simulink model "RL_Runcontrol"  (R2024b)
settings: Solver=VariableStepAuto  StartTime=0.0  StopTime=60  RelTol=1e-3
libraries: simulink x2, rllib x1, Solver_SF x1
settings Model: Creator=Administrator  LastModifiedBy=Administrator

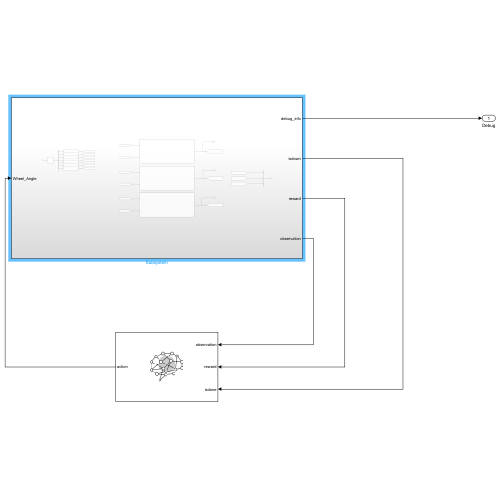
[thumbnail: Simulink's stored preview of the top-level diagram]
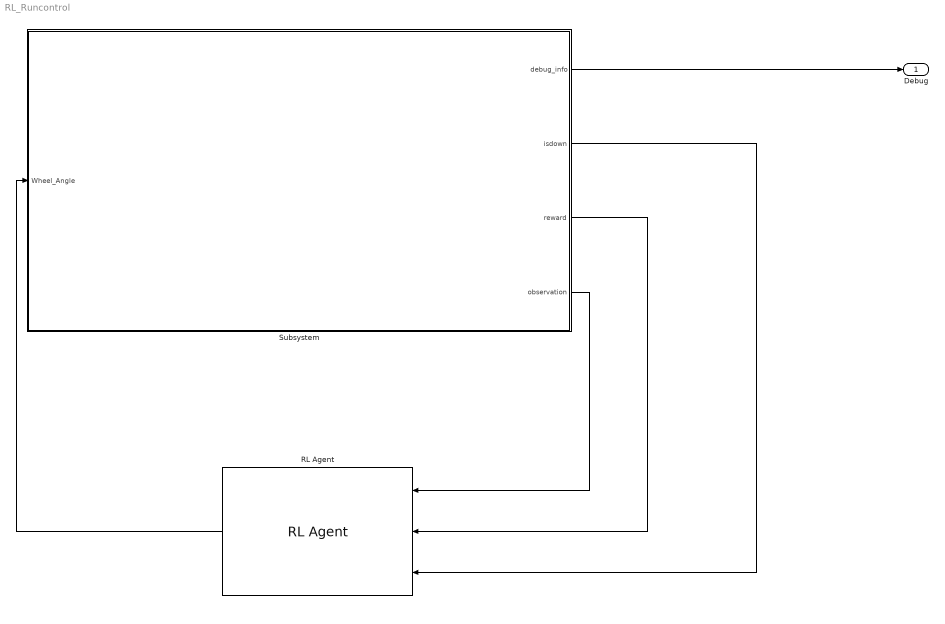
== system RL_Runcontrol ==
  RL Agent : rllib/RL Agent  Agent=agent  ExternalActionAsInput=off  ProvideLastAction=off  ProvideCumRwd=off  TreatAsDirectFeedthrough=on  UseStrictObservationDataTypes=off
  Subsystem : Subsystem
  Debug : Outport
  wires:
  RL Agent/1 -> Subsystem/1(Wheel_Angle)
  Subsystem/4(observation) -> RL Agent/1
  Subsystem/3(reward) -> RL Agent/2
  Subsystem/2(isdown) -> RL Agent/3
  Subsystem/1(debug_info) -> Debug/1

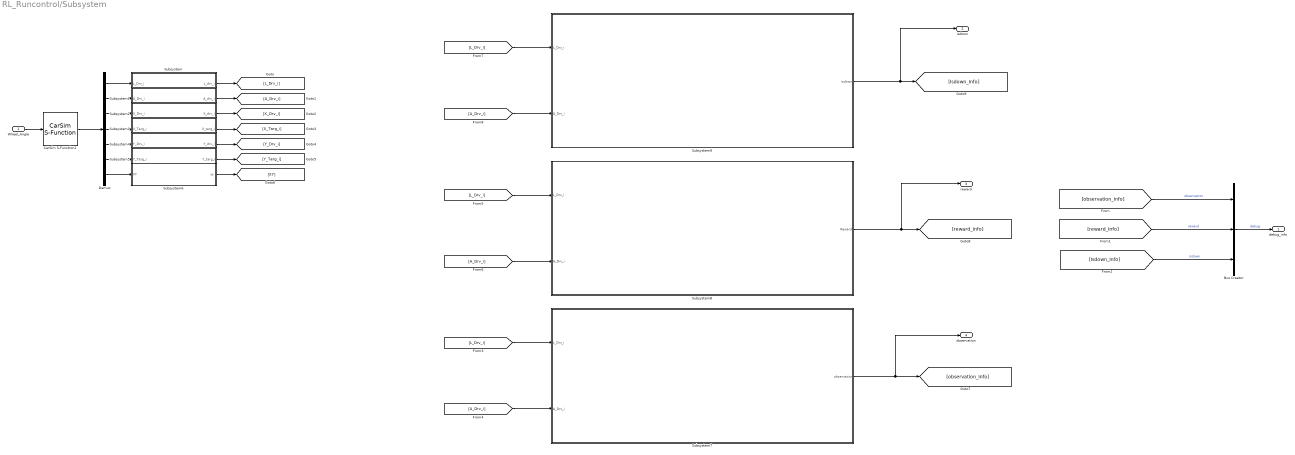
== system RL_Runcontrol/Subsystem ==
  Wheel_Angle : Inport
  Bus Creator : BusCreator  Inputs=3
  CarSim S-Function1 : Solver_SF/CarSim S-Function  Priority=1  SIMFILE=simfile.sim  Run_RTs=off  vs_state_ind=Run  StopMode_ind=Vehicle Model
  Demux : Demux  Outputs=[3 3 3 3 3 3 2]
  Subsystem : Subsystem
  Subsystem1 : Subsystem
  Subsystem2 : Subsystem
  Subsystem3 : Subsystem
  Subsystem4 : Subsystem
  Subsystem5 : Subsystem
  Subsystem6 : Subsystem
  Subsystem7 : Subsystem
  Subsystem8 : Subsystem
  Subsystem9 : Subsystem
  debug_info : Outport
  isdown : Outport  Port=2
  reward : Outport  Port=3
  observation : Outport  Port=4
  wires:
  CarSim S-Function1/1 -> Demux/1
  Wheel_Angle/1 -> CarSim S-Function1/1
  Demux/1 -> Subsystem/1(L_Drv_i)
  Demux/2 -> Subsystem1/1(A_Drv_i)
  Demux/3 -> Subsystem2/1(X_Drv_i)
  Demux/4 -> Subsystem3/1(X_Targ_i)
  Demux/5 -> Subsystem4/1(Y_Drv_i)
  Demux/6 -> Subsystem5/1(Y_Targ_i)
  Demux/7 -> Subsystem6/1(XY)
  Subsystem/1(L_drv_i) -> [L_Drv_i]
  Subsystem1/1(A_drv_i) -> [A_Drv_i]
  Subsystem2/1(X_drv_i) -> [X_Drv_i]
  Subsystem3/1(X_targ_i) -> [X_Targ_i]
  Subsystem4/1(Y_drv_i) -> [Y_Drv_i]
  Subsystem5/1(Y_targ_i) -> [Y_Targ_i]
  Subsystem6/1(xy) -> [XY]
  Subsystem7/1(observation) -> observation/1, [observation_Info]
  Subsystem8/1(Reward) -> reward/1, [reward_Info]
  Subsystem9/1(isdown) -> isdown/1, [Isdown_Info]
  [Isdown_Info] -> Bus Creator/3  "isdown"
  [reward_Info] -> Bus Creator/2  "reward"
  [observation_Info] -> Bus Creator/1  "observation"
  Bus Creator/1 -> debug_info/1  "debug"
  [L_Drv_i] -> Subsystem7/1(L_Drv_i)
  [A_Drv_i] -> Subsystem7/2(A_Drv_i)
  [A_Drv_i] -> Subsystem8/2(A_Drv_i)
  [L_Drv_i] -> Subsystem8/1(L_Drv_i)
  [L_Drv_i] -> Subsystem9/1(L_Drv_i)
  [A_Drv_i] -> Subsystem9/2(A_Drv_i)

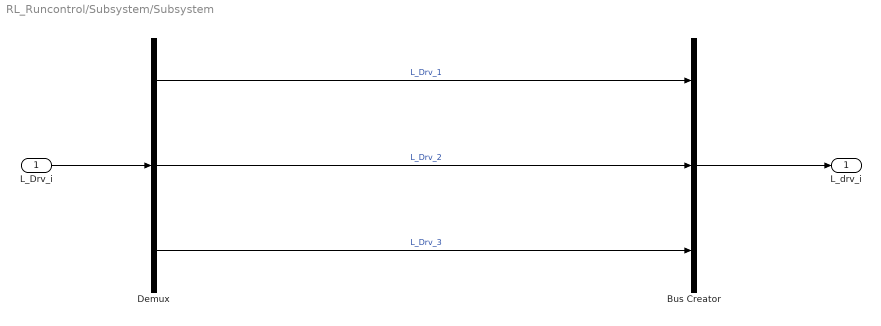
== system RL_Runcontrol/Subsystem/Subsystem ==
  L_Drv_i : Inport
  Bus Creator : BusCreator  Inputs=3
  Demux : Demux  Outputs=3
  L_drv_i : Outport
  wires:
  L_Drv_i/1 -> Demux/1
  Demux/3 -> Bus Creator/3  "L_Drv_3"
  Demux/2 -> Bus Creator/2  "L_Drv_2"
  Demux/1 -> Bus Creator/1  "L_Drv_1"
  Bus Creator/1 -> L_drv_i/1

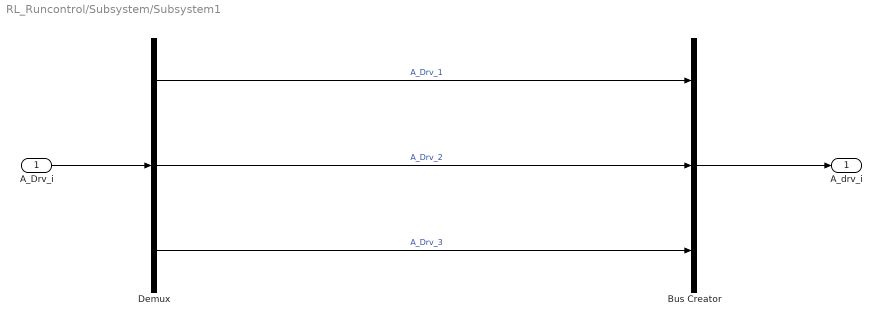
== system RL_Runcontrol/Subsystem/Subsystem1 ==
  A_Drv_i : Inport
  Bus Creator : BusCreator  Inputs=3
  Demux : Demux  Outputs=3
  A_drv_i : Outport
  wires:
  Bus Creator/1 -> A_drv_i/1
  Demux/1 -> Bus Creator/1  "A_Drv_1"
  Demux/2 -> Bus Creator/2  "A_Drv_2"
  Demux/3 -> Bus Creator/3  "A_Drv_3"
  A_Drv_i/1 -> Demux/1

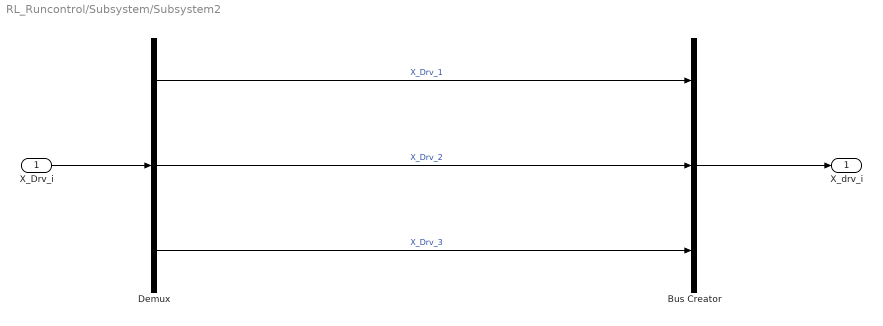
== system RL_Runcontrol/Subsystem/Subsystem2 ==
  X_Drv_i : Inport
  Bus Creator : BusCreator  Inputs=3
  Demux : Demux  Outputs=3
  X_drv_i : Outport
  wires:
  X_Drv_i/1 -> Demux/1
  Demux/3 -> Bus Creator/3  "X_Drv_3"
  Demux/2 -> Bus Creator/2  "X_Drv_2"
  Demux/1 -> Bus Creator/1  "X_Drv_1"
  Bus Creator/1 -> X_drv_i/1

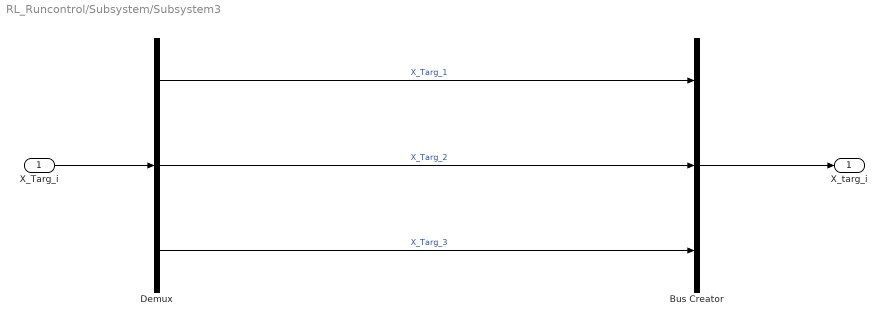
== system RL_Runcontrol/Subsystem/Subsystem3 ==
  X_Targ_i : Inport
  Bus Creator : BusCreator  Inputs=3
  Demux : Demux  Outputs=3
  X_targ_i : Outport
  wires:
  Bus Creator/1 -> X_targ_i/1
  Demux/1 -> Bus Creator/1  "X_Targ_1"
  Demux/2 -> Bus Creator/2  "X_Targ_2"
  Demux/3 -> Bus Creator/3  "X_Targ_3"
  X_Targ_i/1 -> Demux/1

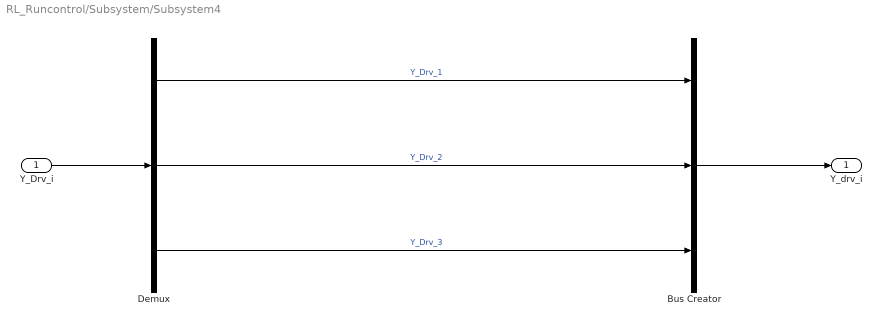
== system RL_Runcontrol/Subsystem/Subsystem4 ==
  Y_Drv_i : Inport
  Bus Creator : BusCreator  Inputs=3
  Demux : Demux  Outputs=3
  Y_drv_i : Outport
  wires:
  Y_Drv_i/1 -> Demux/1
  Demux/3 -> Bus Creator/3  "Y_Drv_3"
  Demux/2 -> Bus Creator/2  "Y_Drv_2"
  Demux/1 -> Bus Creator/1  "Y_Drv_1"
  Bus Creator/1 -> Y_drv_i/1

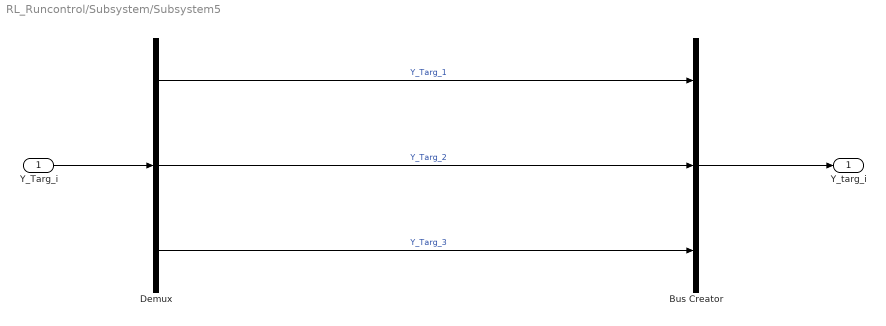
== system RL_Runcontrol/Subsystem/Subsystem5 ==
  Y_Targ_i : Inport
  Bus Creator : BusCreator  Inputs=3
  Demux : Demux  Outputs=3
  Y_targ_i : Outport
  wires:
  Bus Creator/1 -> Y_targ_i/1
  Demux/1 -> Bus Creator/1  "Y_Targ_1"
  Demux/2 -> Bus Creator/2  "Y_Targ_2"
  Demux/3 -> Bus Creator/3  "Y_Targ_3"
  Y_Targ_i/1 -> Demux/1

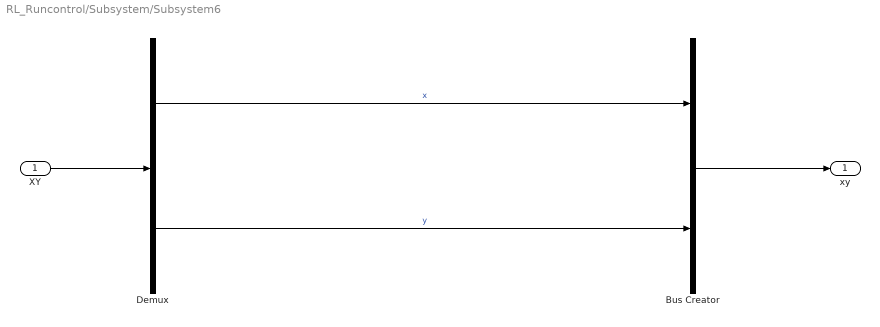
== system RL_Runcontrol/Subsystem/Subsystem6 ==
  XY : Inport
  Bus Creator : BusCreator  Inputs=2
  Demux : Demux  Outputs=2
  xy : Outport
  wires:
  XY/1 -> Demux/1
  Demux/2 -> Bus Creator/2  "y"
  Demux/1 -> Bus Creator/1  "x"
  Bus Creator/1 -> xy/1

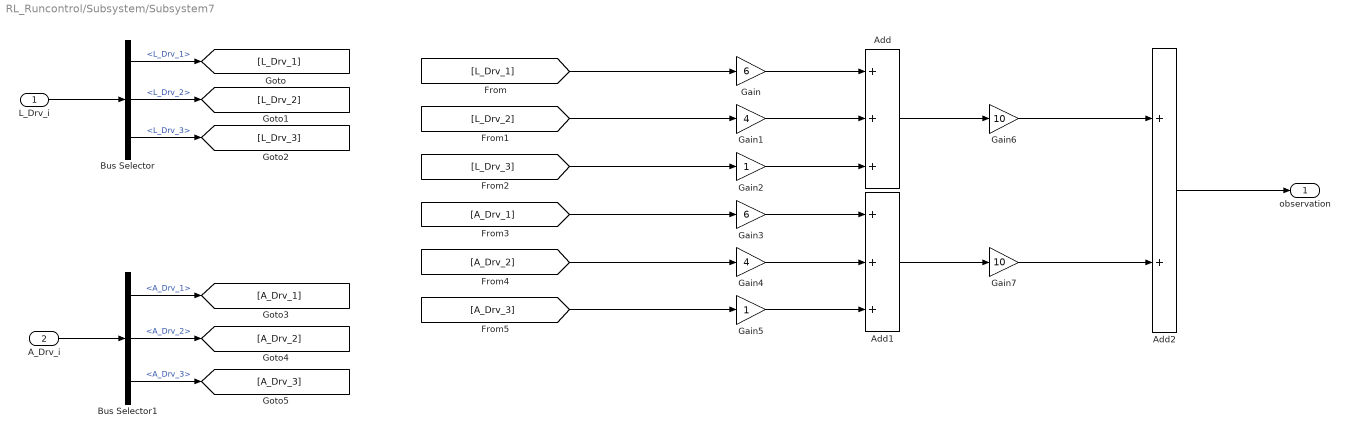
== system RL_Runcontrol/Subsystem/Subsystem7 ==
  L_Drv_i : Inport
  A_Drv_i : Inport  Port=2
  Add : Sum  Inputs=+++
  Add1 : Sum  Inputs=+++
  Add2 : Sum
  Bus Selector : BusSelector  OutputSignals=L_Drv_1,L_Drv_2,L_Drv_3
  Bus Selector1 : BusSelector  OutputSignals=A_Drv_1,A_Drv_2,A_Drv_3
  Gain : Gain  Gain=6
  Gain1 : Gain  Gain=4
  Gain2 : Gain
  Gain3 : Gain  Gain=6
  Gain4 : Gain  Gain=4
  Gain5 : Gain
  Gain6 : Gain  Gain=10
  Gain7 : Gain  Gain=10
  observation : Outport
  wires:
  L_Drv_i/1 -> Bus Selector/1
  A_Drv_i/1 -> Bus Selector1/1
  Bus Selector/1 -> [L_Drv_1]  "<L_Drv_1>"
  Bus Selector/2 -> [L_Drv_2]  "<L_Drv_2>"
  Bus Selector/3 -> [L_Drv_3]  "<L_Drv_3>"
  Bus Selector1/1 -> [A_Drv_1]  "<A_Drv_1>"
  Bus Selector1/2 -> [A_Drv_2]  "<A_Drv_2>"
  Bus Selector1/3 -> [A_Drv_3]  "<A_Drv_3>"
  [L_Drv_1] -> Gain/1
  [L_Drv_2] -> Gain1/1
  [L_Drv_3] -> Gain2/1
  [A_Drv_1] -> Gain3/1
  [A_Drv_2] -> Gain4/1
  [A_Drv_3] -> Gain5/1
  Gain/1 -> Add/1
  Gain1/1 -> Add/2
  Gain2/1 -> Add/3
  Gain3/1 -> Add1/1
  Gain4/1 -> Add1/2
  Gain5/1 -> Add1/3
  Add/1 -> Gain6/1
  Add1/1 -> Gain7/1
  Gain6/1 -> Add2/1
  Gain7/1 -> Add2/2
  Add2/1 -> observation/1

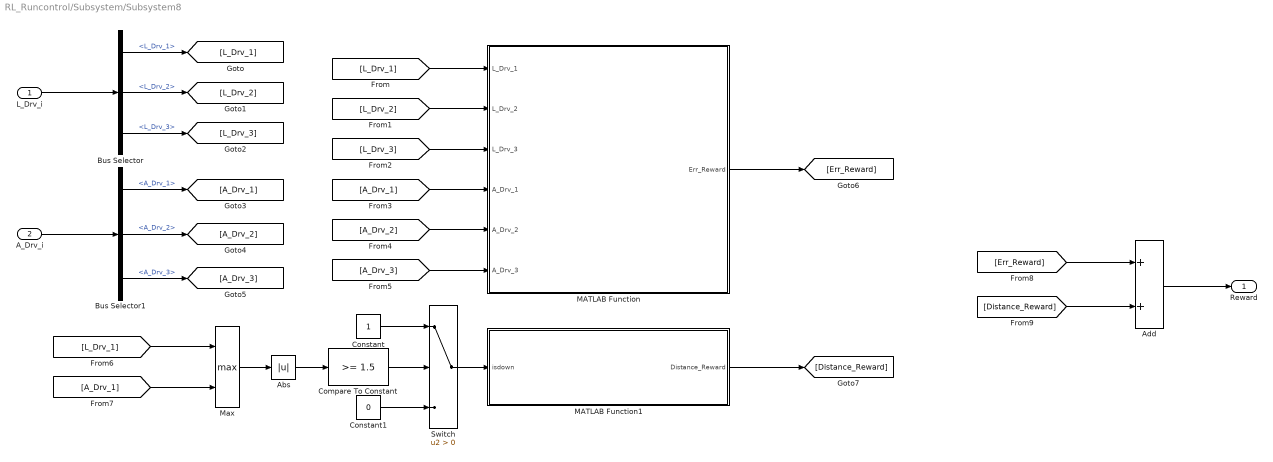
== system RL_Runcontrol/Subsystem/Subsystem8 ==
  L_Drv_i : Inport
  A_Drv_i : Inport  Port=2
  Abs : Abs  SaturateOnIntegerOverflow=off
  Add : Sum
  Bus Selector : BusSelector  OutputSignals=L_Drv_1,L_Drv_2,L_Drv_3
  Bus Selector1 : BusSelector  OutputSignals=A_Drv_1,A_Drv_2,A_Drv_3
  Compare To Constant : simulink/Logic and Bit Operations/Compare To Constant  relop=>=  const=1.5  OutDataTypeStr=boolean
  Constant : Constant  OutDataTypeStr=boolean
  Constant1 : Constant  Value=0  OutDataTypeStr=boolean
  MATLAB Function : MATLAB Function  TreatAsAtomicUnit=on
  MATLAB Function1 : MATLAB Function  TreatAsAtomicUnit=on
  Max : MinMax  Function=max  Inputs=2
  Switch : Switch  Criteria=u2 > Threshold  SaturateOnIntegerOverflow=off  InputSameDT=off
  Reward : Outport
  wires:
  L_Drv_i/1 -> Bus Selector/1
  A_Drv_i/1 -> Bus Selector1/1
  Bus Selector/1 -> [L_Drv_1]  "<L_Drv_1>"
  Bus Selector/2 -> [L_Drv_2]  "<L_Drv_2>"
  Bus Selector/3 -> [L_Drv_3]  "<L_Drv_3>"
  Bus Selector1/1 -> [A_Drv_1]  "<A_Drv_1>"
  Bus Selector1/2 -> [A_Drv_2]  "<A_Drv_2>"
  Bus Selector1/3 -> [A_Drv_3]  "<A_Drv_3>"
  [L_Drv_1] -> MATLAB Function/1(L_Drv_1)
  [L_Drv_2] -> MATLAB Function/2(L_Drv_2)
  [L_Drv_3] -> MATLAB Function/3(L_Drv_3)
  [A_Drv_1] -> MATLAB Function/4(A_Drv_1)
  [A_Drv_2] -> MATLAB Function/5(A_Drv_2)
  [A_Drv_3] -> MATLAB Function/6(A_Drv_3)
  MATLAB Function/1(Err_Reward) -> [Err_Reward]
  MATLAB Function1/1(Distance_Reward) -> [Distance_Reward]
  Constant1/1 -> Switch/3
  Switch/1 -> MATLAB Function1/1(isdown)
  Constant/1 -> Switch/1
  Compare To Constant/1 -> Switch/2
  Abs/1 -> Compare To Constant/1
  Max/1 -> Abs/1
  [L_Drv_1] -> Max/1
  [A_Drv_1] -> Max/2
  [Err_Reward] -> Add/1
  [Distance_Reward] -> Add/2
  Add/1 -> Reward/1

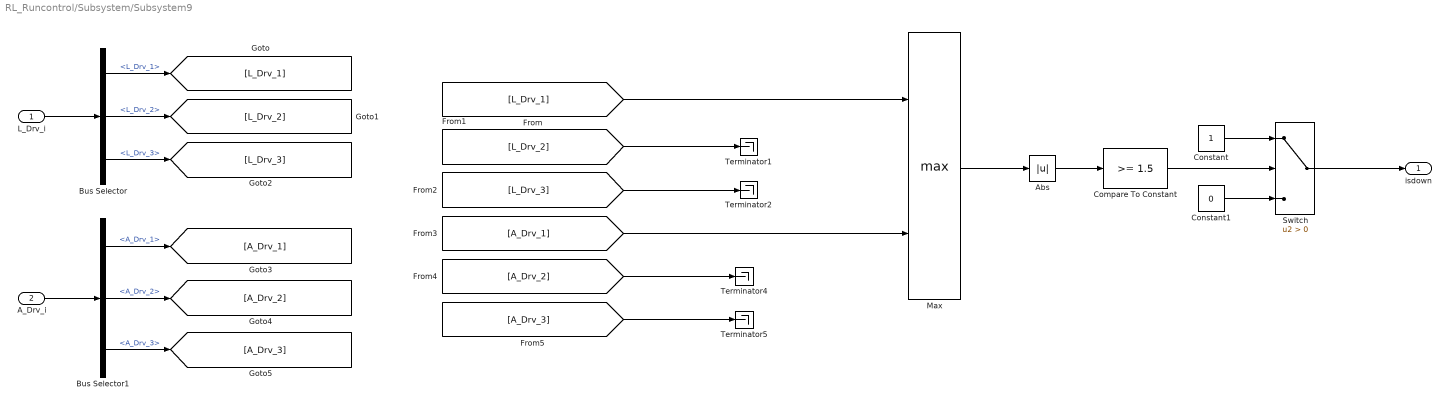
== system RL_Runcontrol/Subsystem/Subsystem9 ==
  L_Drv_i : Inport
  A_Drv_i : Inport  Port=2
  Abs : Abs  SaturateOnIntegerOverflow=off
  Bus Selector : BusSelector  OutputSignals=L_Drv_1,L_Drv_2,L_Drv_3
  Bus Selector1 : BusSelector  OutputSignals=A_Drv_1,A_Drv_2,A_Drv_3
  Compare To Constant : simulink/Logic and Bit Operations/Compare To Constant  relop=>=  const=1.5  OutDataTypeStr=boolean
  Constant : Constant  OutDataTypeStr=boolean
  Constant1 : Constant  Value=0  OutDataTypeStr=boolean
  Max : MinMax  Function=max  Inputs=2
  Switch : Switch  Criteria=u2 > Threshold  SaturateOnIntegerOverflow=off  InputSameDT=off
  Terminator{1..2,4..5} (4 alike) : Terminator
  isdown : Outport
  wires:
  L_Drv_i/1 -> Bus Selector/1
  A_Drv_i/1 -> Bus Selector1/1
  Bus Selector/1 -> [L_Drv_1]  "<L_Drv_1>"
  Bus Selector/2 -> [L_Drv_2]  "<L_Drv_2>"
  Bus Selector/3 -> [L_Drv_3]  "<L_Drv_3>"
  Bus Selector1/1 -> [A_Drv_1]  "<A_Drv_1>"
  Bus Selector1/2 -> [A_Drv_2]  "<A_Drv_2>"
  Bus Selector1/3 -> [A_Drv_3]  "<A_Drv_3>"
  [L_Drv_1] -> Max/1
  [L_Drv_2] -> Terminator1/1
  [L_Drv_3] -> Terminator2/1
  [A_Drv_1] -> Max/2
  [A_Drv_2] -> Terminator4/1
  [A_Drv_3] -> Terminator5/1
  Max/1 -> Abs/1
  Abs/1 -> Compare To Constant/1
  Compare To Constant/1 -> Switch/2
  Constant/1 -> Switch/1
  Constant1/1 -> Switch/3
  Switch/1 -> isdown/1

== matlab function RL_Runcontrol/Subsystem/Subsystem8/MATLAB Function1 ==
  data: isdown input; Distance_Reward output
function Distance_Reward = fcn(isdown)

cot = 0;
if isdown == 0
    cot = cot + 1;
    Distance_Reward = cot;
else
    Distance_Reward = -100;
end
end

== matlab function RL_Runcontrol/Subsystem/Subsystem8/MATLAB Function ==
  data: Err_Reward output; L_Drv_1 input; L_Drv_2 input; L_Drv_3 input; A_Drv_1 input; A_Drv_2 input; A_Drv_3 input
function Err_Reward = fcn(L_Drv_1, L_Drv_2, L_Drv_3, A_Drv_1, A_Drv_2, A_Drv_3)

L_Err_Reward = -(L_Drv_1 + L_Drv_2 + L_Drv_3);
A_Err_Reward = -(A_Drv_1 + A_Drv_2 + A_Drv_3);
Err_Reward = L_Err_Reward + A_Err_Reward;
end
